simulink model "Problem_1_Part_A"  (R2018b)
settings: Solver=FixedStepAuto  StartTime=0.0  StopTime=600  FixedStep=0.002  RelTol=1e-3
InitFcn:
  | Initial_Data
StopFcn:
  | Plots_Problme_1_Part_A
values from neighbouring files (symbols this model uses):
  Gamma0 = 0.3446    [Initial_Data.m]    (also in Secant_Method.m = ((Gamma_max + Gamma_min)/2))
  GM = 3.986004418*(10^14)    (= 398600441800000)    [Initial_Data.m]    (also in Secant_Method.m)
  Long0 = 25    [Initial_Data.m]    (also in Secant_Method.m)
  R0 = 6371000    [Initial_Data.m]    (also in Secant_Method.m)
  V0 = 5193    [Initial_Data.m]    (also in Secant_Method.m = sqrt( (GM*( 1-cos(Phi)))/((R0*cos(Gamma0))*((R0*cos(Gamma0)))
settings Model: Creator=User  LastModifiedBy=User

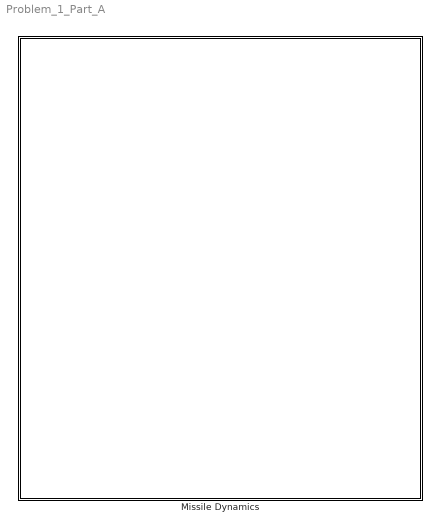
== system Problem_1_Part_A ==
  Missile Dynamics : Subsystem

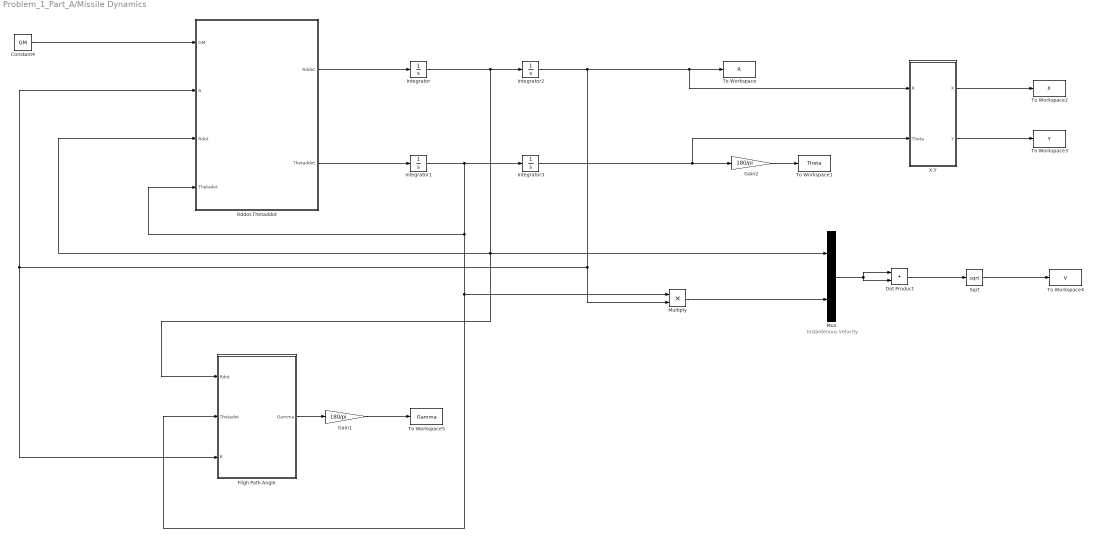
== system Problem_1_Part_A/Missile Dynamics ==
  note: Instantenous Velocity
  Constant4 : Constant  Value=GM
  Dot Product : DotProduct  InputSameDT=on  OutDataTypeStr=Inherit: Inherit via internal rule
  Fligh Path Angle : MATLAB Function  TreatAsAtomicUnit=on
  Gain1 : Gain  Gain=180/pi
  Gain2 : Gain  Gain=180/pi
  Integrator : Integrator  InitialCondition=V0*sin(Gamma0)
  Integrator1 : Integrator  InitialCondition=(V0*cos(Gamma0))/R0
  Integrator2 : Integrator  InitialCondition=R0
  Integrator3 : Integrator  InitialCondition=Long0*pi/180
  Multiply : Product
  Mux : Mux  Inputs=2
  Rddot,Thetaddot : MATLAB Function  TreatAsAtomicUnit=on
  Sqrt : Sqrt  SaturateOnIntegerOverflow=on
  To Workspace : ToWorkspace  VariableName=R  SaveFormat=Timeseries  SampleTime=-1
  To Workspace1 : ToWorkspace  VariableName=Theta  SaveFormat=Timeseries  SampleTime=-1
  To Workspace2 : ToWorkspace  VariableName=X  SaveFormat=Timeseries  SampleTime=-1
  To Workspace3 : ToWorkspace  VariableName=Y  SaveFormat=Timeseries  SampleTime=-1
  To Workspace4 : ToWorkspace  VariableName=V  SaveFormat=Timeseries  SampleTime=-1
  To Workspace5 : ToWorkspace  VariableName=Gamma  SaveFormat=Timeseries  SampleTime=-1
  X,Y : MATLAB Function  TreatAsAtomicUnit=on
  wires:
  Rddot,Thetaddot/2(Thetaddot) -> Integrator1/1
  Rddot,Thetaddot/1(Rddot) -> Integrator/1
  Integrator/1 -> Mux/1, Rddot,Thetaddot/3(Rdot), Fligh Path Angle/1(Rdot), Integrator2/1
  Integrator1/1 -> Integrator3/1, Multiply/1, Fligh Path Angle/2(Thetadot), Rddot,Thetaddot/4(Thetadot)
  Integrator3/1 -> Gain2/1, X,Y/2(Theta)
  Integrator2/1 -> Multiply/2, Fligh Path Angle/3(R), Rddot,Thetaddot/2(R), X,Y/1(R), To Workspace/1
  X,Y/1(X) -> To Workspace2/1
  X,Y/2(Y) -> To Workspace3/1
  Constant4/1 -> Rddot,Thetaddot/1(GM)
  Sqrt/1 -> To Workspace4/1
  Fligh Path Angle/1(Gamma) -> Gain1/1
  Dot Product/1 -> Sqrt/1
  Mux/1 -> Dot Product/1, Dot Product/2
  Gain1/1 -> To Workspace5/1
  Multiply/1 -> Mux/2
  Gain2/1 -> To Workspace1/1

== matlab function Problem_1_Part_A/Missile Dynamics/Fligh Path Angle ==
  data: Rdot input; Gamma output; Thetadot input; R input
function Gamma = fcn(Rdot,Thetadot,R)

Gamma = atan((Rdot)/(R*Thetadot));

== matlab function Problem_1_Part_A/Missile Dynamics/X,Y ==
  data: R input; X output; Theta input; Y output
function [X,Y] = fcn(R,Theta)

X = R*cos(Theta);
Y = R*sin(Theta);

== matlab function Problem_1_Part_A/Missile Dynamics/Rddot,Thetaddot ==
  data: GM input; Rddot output; R input; Rdot input; Thetadot input; Thetaddot output
function [Rddot,Thetaddot]  = fcn(GM,R,Rdot,Thetadot)

Rddot = R*Thetadot^2 - (GM)/(R^2);
Thetaddot = (-2*Rdot*Thetadot)/(R);
